simulink model "untitled"  (R2021a)
settings: Solver=ode1  StartTime=0.0  StopTime=inf  FixedStep=0.005  RelTol=1e-3
libraries: qbmove_library x2, dspswit3 x1
settings Model: Creator=mgnocco  LastModifiedBy=mgnocco

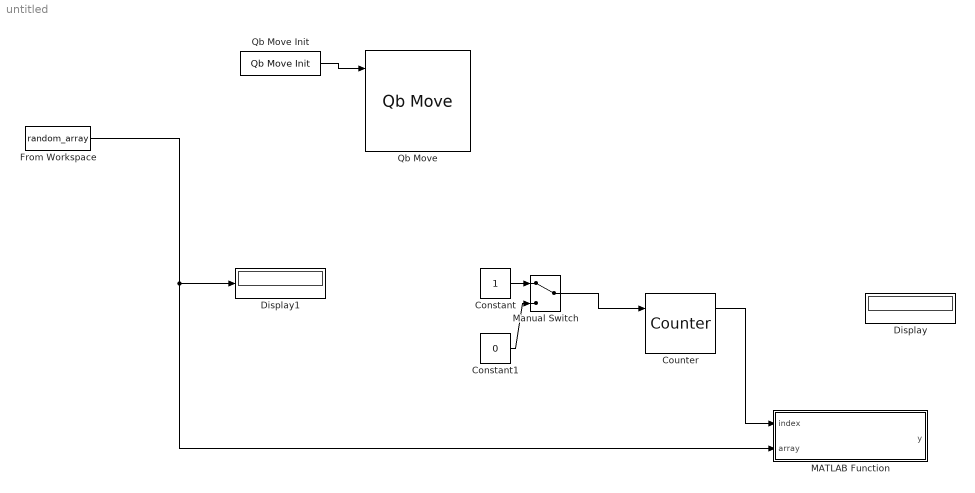
== system untitled ==
  Constant : Constant
  Constant1 : Constant  Value=0
  Counter : dspswit3/Counter  Direction=Up  CountEvent=Rising edge  CounterSize=User defined  MaxCount=255  InitialCount=0  Output=Count and Hit  HitValue=32  ResetInput=on  SamplesPerFrame=1  Ts=1  CntDtype=double  HitDtype=Logical
  Display : Display
  Display1 : Display
  From Workspace : FromWorkspace  VariableName=random_array
  MATLAB Function : MATLAB Function  TreatAsAtomicUnit=on
  Manual Switch : ManualSwitch
  Qb Move : qbmove_library/Qb Move  ID=1  ACTIVE_COMM_DIRECTIONS=Both  CONTROL_MODE=Prime Movers Positions  DAISY_CHAINING=off  MAX_ANG=0  SW_LIMIT=inf  OFFSET=0  ACTIVATE=on  WDT=0.0  UNIT=Degrees
      settings: SourceProductName=Qb Move Library
  Qb Move Init : qbmove_library/Qb Move Init  NUMBER_OF_COM='COM7'  BAUD_RATE_COM=2000000
      settings: SourceProductName=Qb Move Library
  wires:
  Qb Move Init/1 -> Qb Move/1
  From Workspace/1 -> Display1/1, MATLAB Function/2(array)
  Manual Switch/1 -> Counter/1
  Constant/1 -> Manual Switch/1
  Constant1/1 -> Manual Switch/2
  Counter/1 -> MATLAB Function/1(index)
  ? -> Display/1

== matlab function untitled/MATLAB Function ==
  data: index input; y output; array input
function y = get_element(index, array)
    % Output the current element from the array
    if index <= length(array)
        y = array(index);
    else
        y = 0;  % Output 0 if index is out of bounds
    end
end
